simulink model "ss1"  (Simulink 7.8)
settings: Solver=ode45  StartTime=0.0  StopTime=0.5  RelTol=1e-3
libraries: powerlib x27
settings Model: Creator=sundeep  LastModifiedBy=sundeep  SimulationMode=accelerator

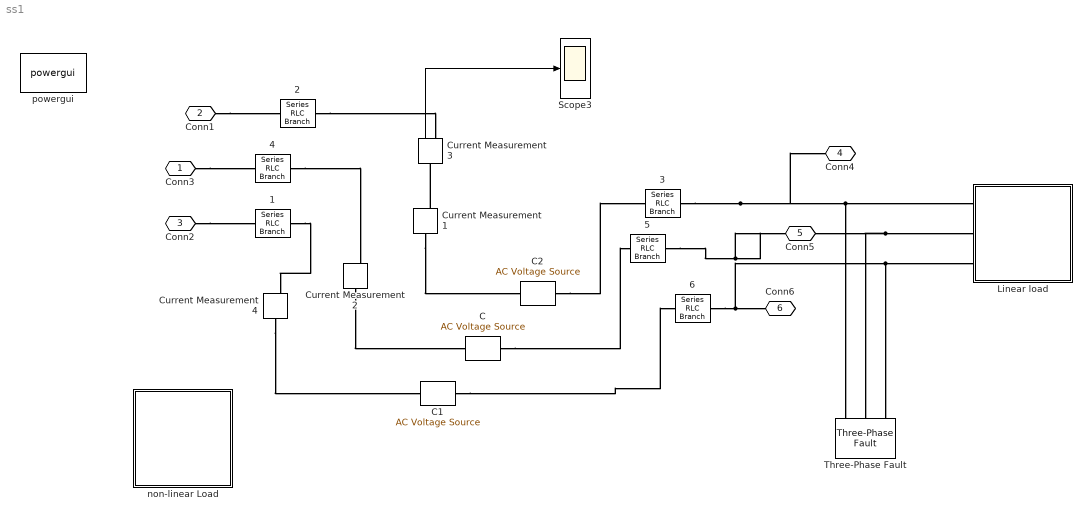
== system ss1 ==
    {1..6} (6 alike) : powerlib/Elements/Series RLC Branch  LConnTagsString=__new0  RConnTagsString=__new0  BranchType=RL  Resistance=0.6  Inductance=(2.5e-3)/2  SetiL0=off  InitialCurrent=0  Capacitance=1e-6  Setx0=off  InitialVoltage=0  Measurements=None
  C : powerlib/Electrical Sources/AC Voltage Source  Amplitude=400*1.414  Phase=-240  Frequency=50  SampleTime=0  Measurements=None
  C1 : powerlib/Electrical Sources/AC Voltage Source  Amplitude=400*1.414  Phase=-240  Frequency=50  SampleTime=0  Measurements=None
  C2 : powerlib/Electrical Sources/AC Voltage Source  Amplitude=400*1.414  Phase=-240  Frequency=50  SampleTime=0  Measurements=None
  Current Measurement{1..4} (4 alike) : powerlib/Measurements/Current Measurement  PhasorSimulation=off  OutputType=Complex  PSBequivalent=0
  Linear load : Subsystem
  Scope3 : Scope
      settings: TimeRange=0.5  YMin=10  YMax=52.5  SaveName=i  SampleInput=on  SampleTime=1e-6
  Three-Phase Fault : powerlib/Elements/Three-Phase Fault  FaultA=on  FaultB=on  FaultC=off  FaultResistance=10  GroundFault=off  GroundResistance=1  External=off  SwitchStatus=[1 0]  SwitchTimes=[ 0.1 0.3]  InitialStates=[0 0 1]  SnubberResistance=1e6  SnubberCapacitance=inf  Measurements=None
  non-linear Load : Subsystem
  powergui : powerlib/powergui  Priority=1  SimulationMode=Continuous  SolverType=Tustin  SampleTime=50e-6  frequency=60  SPID=off  DisableSnubberDevices=off  DisableRonSwitches=off  DisableVfSwitches=off  SwTol=0  Interpol=off  DisplayEquations=off  FunctionMessages=off  frequencyindice=0  Pbase=100e6  ErrMax=1e-4  Iterations=50  UnitsV=kV  UnitsW=MW  echomessages=off  HookPort=off  EnableUseOfTLC=off  x0status=blocks  RestoreLinks=warning  ResistiveCurrentMeasurement=off  Ylog=off  Xlog=on  ShowGrid=off  save=off  variable=ZData  ZoomFFT=off  StartTime=0.0  cycles=1  DisplayStyle=1  FreqAxis=off  MaxFrequency=1000  frequencyindicesteady=1  display=off  methode=off
  Conn3 : PMIOPort  Port=1  Side=Left
  Conn1 : PMIOPort  Port=2  Side=Right
  Conn2 : PMIOPort  Port=3  Side=Left
  Conn4 : PMIOPort  Port=4  Side=Right
  Conn5 : PMIOPort  Port=5  Side=Left
  Conn6 : PMIOPort  Port=6  Side=Right
  wires:
  Current Measurement3/1 -> Scope3/1
  connections:
  Conn1/RConn1 -- "  2"/RConn1
  Conn3/RConn1 -- "  4"/RConn1
  Conn2/RConn1 -- "  1"/RConn1
  "  2"/LConn1 -- Current Measurement3/RConn1
  "  4"/LConn1 -- Current Measurement2/RConn1
  "  1"/LConn1 -- Current Measurement4/RConn1
  Current Measurement1/RConn1 -- Current Measurement3/LConn1
  Current Measurement2/LConn1 -- C/RConn1
  Current Measurement4/LConn1 -- C1/RConn1
  Current Measurement1/LConn1 -- C2/RConn1
  C2/LConn1 -- "  3"/RConn1
  C/LConn1 -- "  5"/RConn1
  C1/LConn1 -- "  6"/RConn1
  "  3"/LConn1 -- Conn4/RConn1 -- Linear load/LConn1 -- Three-Phase Fault/LConn1
  "  5"/LConn1 -- Conn5/RConn1 -- Linear load/LConn2 -- Three-Phase Fault/LConn2
  "  6"/LConn1 -- Conn6/RConn1 -- Linear load/LConn3 -- Three-Phase Fault/LConn3

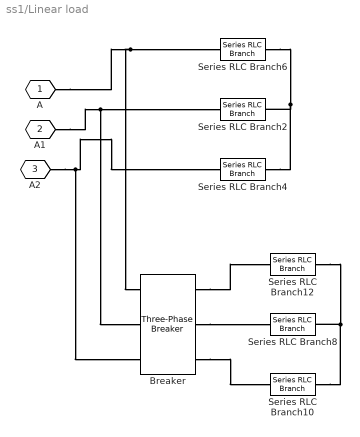
== system ss1/Linear load ==
  Breaker : powerlib/Elements/Three-Phase Breaker  InitialState=open  SwitchA=on  SwitchB=on  SwitchC=on  SwitchTimes=[0.2 0.4]  External=off  BreakerResistance=0.001  SnubberResistance=1e6  SnubberCapacitance=inf  Measurements=None
  Series RLC Branch{2,4,6,8,10,12} (6 alike) : powerlib/Elements/Series RLC Branch  LConnTagsString=__new0  RConnTagsString=__new0  BranchType=R  Resistance=30  Inductance=1.0  SetiL0=off  InitialCurrent=0  Capacitance=1.0  Setx0=off  InitialVoltage=0  Measurements=None
  A : PMIOPort  Tag=PMCPort  Port=1  Side=Left
  A1 : PMIOPort  Tag=PMCPort  Port=2  Side=Left
  A2 : PMIOPort  Tag=PMCPort  Port=3  Side=Left
  connections:
  A/RConn1 -- Series RLC Branch6/LConn1 -- Breaker/LConn1
  A1/RConn1 -- Series RLC Branch2/LConn1 -- Breaker/LConn2
  A2/RConn1 -- Series RLC Branch4/LConn1 -- Breaker/LConn3
  Breaker/RConn1 -- Series RLC Branch12/LConn1
  Breaker/RConn2 -- Series RLC Branch8/LConn1
  Breaker/RConn3 -- Series RLC Branch10/LConn1
  Series RLC Branch6/RConn1 -- Series RLC Branch2/RConn1 -- Series RLC Branch4/RConn1
  Series RLC Branch12/RConn1 -- Series RLC Branch8/RConn1 -- Series RLC Branch10/RConn1

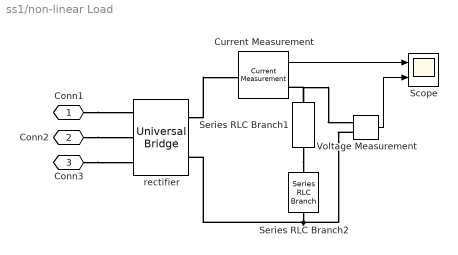
== system ss1/non-linear Load ==
  Current Measurement : powerlib/Measurements/Current Measurement  PhasorSimulation=off  OutputType=Complex  PSBequivalent=0
  Scope : Scope  NumInputPorts=2
      settings: YMin=0~0  YMax=110~750  SaveName=ScopeData6
  Series RLC Branch1 : powerlib/Elements/Series RLC Branch  LConnTagsString=__new0  RConnTagsString=__new0  BranchType=R  Resistance=30  Inductance=1.0  SetiL0=off  InitialCurrent=0  Capacitance=1.0  Setx0=off  InitialVoltage=0  Measurements=None
  Series RLC Branch2 : powerlib/Elements/Series RLC Branch  LConnTagsString=__new0  RConnTagsString=__new0  BranchType=L  Resistance=1.0  Inductance=100e-3  SetiL0=off  InitialCurrent=0  Capacitance=1.0  Setx0=off  InitialVoltage=0  Measurements=None
  Voltage Measurement : powerlib/Measurements/Voltage Measurement  PhasorSimulation=off  OutputType=Complex  PSBequivalent=0
  rectifier : powerlib/Power Electronics/Universal Bridge  Arms=3  SnubberResistance=1e5  SnubberCapacitance=1e-6  Device=Diodes  Ron=1e-3  Lon=0  ForwardVoltages="[  0  0  ]"  ForwardVoltage=0  GTOparameters=[ 10e-6 , 20e-6 ]  IGBTparameters=[ 1e-6 , 2e-6 ]  Measurements=None  Measurements_2=None  converterType=Rectifier
  Conn1 : PMIOPort  Port=1  Side=Left
  Conn2 : PMIOPort  Port=2  Side=Left
  Conn3 : PMIOPort  Port=3  Side=Left
  wires:
  Voltage Measurement/1 -> Scope/2
  Current Measurement/1 -> Scope/1
  connections:
  Voltage Measurement/LConn2 -- rectifier/RConn2 -- Series RLC Branch2/RConn1
  Conn1/RConn1 -- rectifier/LConn1
  Conn2/RConn1 -- rectifier/LConn2
  Conn3/RConn1 -- rectifier/LConn3
  rectifier/RConn1 -- Current Measurement/LConn1
  Series RLC Branch1/LConn1 -- Current Measurement/RConn1 -- Voltage Measurement/LConn1
  Series RLC Branch1/RConn1 -- Series RLC Branch2/LConn1
